simulink model "bh_tmp_model_for_lagr"  (R2016b)
settings: Solver=VariableStepAuto  StartTime=0.0  StopTime=10.0  RelTol=1e-3
settings Model: Creator=bhorton  LastModifiedBy=bhorton

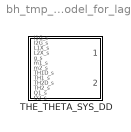
== system bh_tmp_model_for_lagr ==
  THE_THETA_SYS_DD : MATLAB Function  TreatAsAtomicUnit=on

== matlab function bh_tmp_model_for_lagr/THE_THETA_SYS_DD ==
  data: I1G_s input; theta1_DD output; I2G_s input; L1X_s input; L2X_s input; g_s input; m1_s input; m2_s input; TH1D_s input; TH1_s input; TH2D_s input; TH2_s input; Q1_s input; Q2_s input; theta2_DD output
function [theta1_DD,theta2_DD] = THE_THETA_SYS_DD(I1G_s,I2G_s,L1X_s,L2X_s,g_s,m1_s,m2_s,TH1D_s,TH1_s,TH2D_s,TH2_s,Q1_s,Q2_s)
%#codegen

%    This function was generated by the Symbolic Math Toolbox version 7.1.
%    13-Feb-2017 14:09:34

theta1_DD = (I2G_s.*Q1_s.*1.6e1-I2G_s.*Q2_s.*1.6e1+L2X_s.^2.*Q1_s.*m2_s.*4.0-L2X_s.^2.*Q2_s.*m2_s.*4.0-L1X_s.*L2X_s.^2.*g_s.*m2_s.^2.*cos(TH1_s).*4.0-L1X_s.*L2X_s.*Q2_s.*m2_s.*cos(TH2_s).*8.0-I2G_s.*L1X_s.*g_s.*m1_s.*cos(TH1_s).*8.0-I2G_s.*L1X_s.*g_s.*m2_s.*cos(TH1_s).*1.6e1+L1X_s.*L2X_s.^3.*TH1D_s.^2.*m2_s.^2.*sin(TH2_s).*2.0+L1X_s.*L2X_s.^3.*TH2D_s.^2.*m2_s.^2.*sin(TH2_s).*2.0+I2G_s.*L1X_s.*L2X_s.*TH1D_s.^2.*m2_s.*sin(TH2_s).*8.0+I2G_s.*L1X_s.*L2X_s.*TH2D_s.^2.*m2_s.*sin(TH2_s).*8.0-L1X_s.*L2X_s.^2.*g_s.*m1_s.*m2_s.*cos(TH1_s).*2.0+L1X_s.*L2X_s.^3.*TH1D_s.*TH2D_s.*m2_s.^2.*sin(TH2_s).*4.0+L1X_s.*L2X_s.^2.*g_s.*m2_s.^2.*cos(TH1_s+TH2_s).*cos(TH2_s).*4.0+L1X_s.^2.*L2X_s.^2.*TH1D_s.^2.*m2_s.^2.*cos(TH2_s).*sin(TH2_s).*4.0+I2G_s.*L1X_s.*L2X_s.*TH1D_s.*TH2D_s.*m2_s.*sin(TH2_s).*1.6e1)./(I1G_s.*I2G_s.*1.6e1+L1X_s.^2.*L2X_s.^2.*m2_s.^2.*4.0+I2G_s.*L1X_s.^2.*m1_s.*4.0+I1G_s.*L2X_s.^2.*m2_s.*4.0+I2G_s.*L1X_s.^2.*m2_s.*1.6e1+L1X_s.^2.*L2X_s.^2.*m1_s.*m2_s-L1X_s.^2.*L2X_s.^2.*m2_s.^2.*cos(TH2_s).^2.*4.0);
if nargout > 1
    theta2_DD = (I1G_s.*Q2_s.*1.6e1-I2G_s.*Q1_s.*1.6e1+I2G_s.*Q2_s.*1.6e1+L1X_s.^2.*Q2_s.*m1_s.*4.0+L1X_s.^2.*Q2_s.*m2_s.*1.6e1-L2X_s.^2.*Q1_s.*m2_s.*4.0+L2X_s.^2.*Q2_s.*m2_s.*4.0-I1G_s.*L2X_s.*g_s.*m2_s.*cos(TH1_s+TH2_s).*8.0+L1X_s.*L2X_s.^2.*g_s.*m2_s.^2.*cos(TH1_s).*4.0-L1X_s.*L2X_s.*Q1_s.*m2_s.*cos(TH2_s).*8.0+L1X_s.*L2X_s.*Q2_s.*m2_s.*cos(TH2_s).*1.6e1+I2G_s.*L1X_s.*g_s.*m1_s.*cos(TH1_s).*8.0+I2G_s.*L1X_s.*g_s.*m2_s.*cos(TH1_s).*1.6e1-L1X_s.*L2X_s.^3.*TH1D_s.^2.*m2_s.^2.*sin(TH2_s).*2.0-L1X_s.^3.*L2X_s.*TH1D_s.^2.*m2_s.^2.*sin(TH2_s).*8.0-L1X_s.*L2X_s.^3.*TH2D_s.^2.*m2_s.^2.*sin(TH2_s).*2.0-L1X_s.^2.*L2X_s.*g_s.*m2_s.^2.*cos(TH1_s+TH2_s).*8.0-L1X_s.^2.*L2X_s.*g_s.*m1_s.*m2_s.*cos(TH1_s+TH2_s).*2.0-I1G_s.*L1X_s.*L2X_s.*TH1D_s.^2.*m2_s.*sin(TH2_s).*8.0-I2G_s.*L1X_s.*L2X_s.*TH1D_s.^2.*m2_s.*sin(TH2_s).*8.0-I2G_s.*L1X_s.*L2X_s.*TH2D_s.^2.*m2_s.*sin(TH2_s).*8.0+L1X_s.*L2X_s.^2.*g_s.*m1_s.*m2_s.*cos(TH1_s).*2.0-L1X_s.*L2X_s.^3.*TH1D_s.*TH2D_s.*m2_s.^2.*sin(TH2_s).*4.0-L1X_s.^3.*L2X_s.*TH1D_s.^2.*m1_s.*m2_s.*sin(TH2_s).*2.0-L1X_s.*L2X_s.^2.*g_s.*m2_s.^2.*cos(TH1_s+TH2_s).*cos(TH2_s).*4.0-L1X_s.^2.*L2X_s.^2.*TH1D_s.^2.*m2_s.^2.*cos(TH2_s).*sin(TH2_s).*8.0-L1X_s.^2.*L2X_s.^2.*TH2D_s.^2.*m2_s.^2.*cos(TH2_s).*sin(TH2_s).*4.0+L1X_s.^2.*L2X_s.*g_s.*m2_s.^2.*cos(TH1_s).*cos(TH2_s).*8.0+L1X_s.^2.*L2X_s.*g_s.*m1_s.*m2_s.*cos(TH1_s).*cos(TH2_s).*4.0-I2G_s.*L1X_s.*L2X_s.*TH1D_s.*TH2D_s.*m2_s.*sin(TH2_s).*1.6e1-L1X_s.^2.*L2X_s.^2.*TH1D_s.*TH2D_s.*m2_s.^2.*cos(TH2_s).*sin(TH2_s).*8.0)./(I1G_s.*I2G_s.*1.6e1+L1X_s.^2.*L2X_s.^2.*m2_s.^2.*4.0+I2G_s.*L1X_s.^2.*m1_s.*4.0+I1G_s.*L2X_s.^2.*m2_s.*4.0+I2G_s.*L1X_s.^2.*m2_s.*1.6e1+L1X_s.^2.*L2X_s.^2.*m1_s.*m2_s-L1X_s.^2.*L2X_s.^2.*m2_s.^2.*cos(TH2_s).^2.*4.0);
end
